simulink model "DIPC"  (R2015a)
settings: Solver=ode1  StartTime=0.0  StopTime=3.0  FixedStep=1e-3  RelTol=1e-3
values from neighbouring files (symbols this model uses):
  deltas = 300    [DIPCinit.m]
  deltav = 2000    [DIPCinit.m]
  ds = 300    [DIPCinit.m]
  dv = 5000    [DIPCinit.m]
  g = [0;0;0]    [DIPCinit.m]
  j0 = 1    [DIPCinit.m]
  j1 = 10    [DIPCinit.m]
  j2 = 10    [DIPCinit.m]
  j3 = 10    [DIPCinit.m]
  j4 = 10    [DIPCinit.m]
  jv = 1    [DIPCinit.m]
  kappas = 500    [DIPCinit.m]
  kappav = 2000    [DIPCinit.m]
  ks = 500    [DIPCinit.m]
  kv = 20000    [DIPCinit.m]
  m0 = 10    [DIPCinit.m]
  m1 = 10    [DIPCinit.m]
  m2 = 10    [DIPCinit.m]
  m3 = 10    [DIPCinit.m]
  m4 = 10    [DIPCinit.m]
  mv = 10    [DIPCinit.m]
libraries: aerolibutil x11, dspinverses x3, aerolibtransform2 x2, simulink x2
settings Model: CovSFcnEnable=off  Creator=Martin  LastModifiedBy=mangerer
settings OptimizationCC: BlockReduction=off  OptimizeBlockIOStorage=off  BufferReuse=off  GlobalBufferReuse=off  ExpressionFolding=off  LocalBlockOutputs=off
settings DebuggingCC: SolverPrmCheckMsg=warning

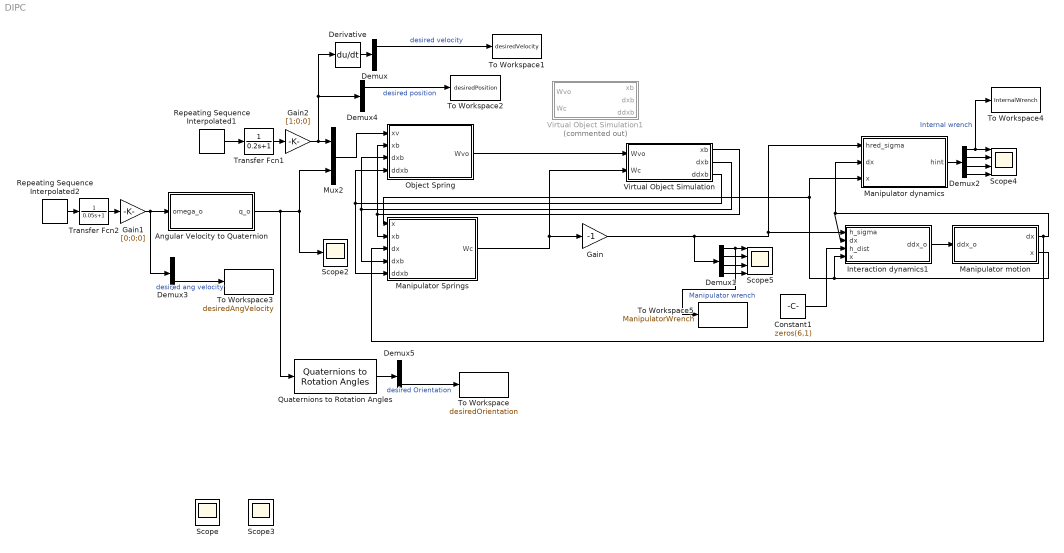
== system DIPC ==
  Angular Velocity to Quaternion : Subsystem
  Constant1 : Constant  Value=zeros(6,1)
  Demux{,3..5} (4 alike) : Demux  Outputs=3
  Demux1 : Demux
  Demux2 : Demux
  Derivative : Derivative
  Gain : Gain  Gain=-1
  Gain1 : Gain  Gain=[0;0;0]
  Gain2 : Gain  Gain=[1;0;0]
  Interaction dynamics1 : Subsystem
  Manipulator Springs : Subsystem
  Manipulator dynamics : Subsystem
  Manipulator motion : Subsystem
  Mux2 : Mux  Inputs=2
  Object Spring : Subsystem
  Quaternions to Rotation Angles : aerolibtransform2/Quaternions to Rotation Angles  rotationOrder=XYZ
  Repeating Sequence Interpolated1 : simulink/Sources/Repeating Sequence Interpolated  OutValues=[0 0 0.5 0.5 1 1 -0.5 -0.5 0 0].'  TimeValues=[0 0.1 0.14 0.9 0.96 1.8 1.95 2.4 2.6 3].'  LookUpMeth=Interpolation-Use End Values  tsamp=0.001  OutMin=[]  OutMax=[]  OutDataTypeStr=double  OutputDataTypeScalingMode=double  OutDataType=fixdt(0,8)  OutScaling=2^-10
  Repeating Sequence Interpolated2 : simulink/Sources/Repeating Sequence Interpolated  OutValues=[0 0 1 1 0 0].'  TimeValues=[0 0.1 1.5 2 2.5 3].'  LookUpMeth=Interpolation-Use End Values  tsamp=0.001  OutMin=[]  OutMax=[]  OutDataTypeStr=double  OutputDataTypeScalingMode=double  OutDataType=fixdt(0,8)  OutScaling=2^-10
  Scope{,3..5} (4 alike) : Scope  NumInputPorts=4
      Scope settings: Floating=on  ShowLegends=on  YMin=-0~0~-30~-0.04  YMax=1.5~1.25~30~0.07  SaveName=ScopeData5
      Scope3 settings: Floating=on  ShowLegends=on  YMin=-0.5~-6~-500~-2e-09  YMax=1~3~700~2.5e-09  SaveName=ScopeData12
      Scope4 settings: ShowLegends=on  YMin=-0.025~-0.025~-0.05~-0.05  YMax=0.05~0.05~0.025~0.025  SaveName=ScopeData6
      Scope5 settings: ShowLegends=on  YMin=-40~-40~-50~-50  YMax=60~60~30~30  SaveName=ScopeData11
  Scope2 : Scope
  To Workspace : ToWorkspace  VariableName=desiredOrientation  SaveFormat=Timeseries  SampleTime=-1
  To Workspace1 : ToWorkspace  VariableName=desiredVelocity  SaveFormat=Timeseries  SampleTime=-1
  To Workspace2 : ToWorkspace  VariableName=desiredPosition  SaveFormat=Timeseries  SampleTime=-1
  To Workspace3 : ToWorkspace  VariableName=desiredAngVelocity  SaveFormat=Timeseries  SampleTime=-1
  To Workspace4 : ToWorkspace  VariableName=InternalWrench  SaveFormat=Timeseries  SampleTime=-1
  To Workspace5 : ToWorkspace  VariableName=ManipulatorWrench  SaveFormat=Timeseries  SampleTime=-1
  Transfer Fcn1 : TransferFcn  Denominator=[0.2 1]
  Transfer Fcn2 : TransferFcn  Denominator=[0.05 1]
  Virtual Object Simulation : Subsystem
  Virtual Object Simulation1 : Subsystem  Commented=on
  wires:
  Object Spring/1(Wvo) -> Virtual Object Simulation/1(Wvo)
  Virtual Object Simulation/1(xb) -> Object Spring/2(xb), Manipulator Springs/2(xb)
  Manipulator Springs/1(Wc) -> Virtual Object Simulation/2(Wc), Gain/1
  Interaction dynamics1/1(ddx_o) -> Manipulator motion/1(ddx_o)
  Constant1/1 -> Interaction dynamics1/3(h_dist)
  Manipulator motion/1(dx) -> Manipulator Springs/3(dx), Manipulator dynamics/2(dx), Interaction dynamics1/2(dx)
  Manipulator motion/2(x) -> Manipulator dynamics/3(x), Manipulator Springs/1(x), Interaction dynamics1/4(x)
  Virtual Object Simulation/2(dxb) -> Manipulator Springs/4(dxb), Object Spring/3(dxb)
  Manipulator dynamics/1(hint) -> Demux2/1
  Demux2/2 -> Scope4/2
  Demux2/4 -> Scope4/4
  Demux2/3 -> Scope4/3
  Demux2/1 -> To Workspace4/1, Scope4/1  "Internal wrench"
  Repeating Sequence Interpolated1/1 -> Transfer Fcn1/1
  Transfer Fcn1/1 -> Gain2/1
  Gain2/1 -> Demux4/1, Derivative/1, Mux2/1
  Mux2/1 -> Object Spring/1(xv)
  Angular Velocity to Quaternion/1(q_o) -> Quaternions to Rotation Angles/1, Mux2/2, Scope2/1
  Repeating Sequence Interpolated2/1 -> Transfer Fcn2/1
  Transfer Fcn2/1 -> Gain1/1
  Gain1/1 -> Demux3/1, Angular Velocity to Quaternion/1(omega_o)
  Gain/1 -> Demux1/1, Manipulator dynamics/1(hred_sigma), Interaction dynamics1/1(h_sigma)
  Demux1/2 -> Scope5/2
  Demux1/4 -> Scope5/4
  Demux1/3 -> Scope5/3
  Demux1/1 -> To Workspace5/1, Scope5/1  "Manipulator wrench"
  Quaternions to Rotation Angles/1 -> Demux5/1
  Demux5/3 -> To Workspace/1  "desired Orientation"
  Demux3/3 -> To Workspace3/1  "desired ang velocity"
  Demux4/1 -> To Workspace2/1  "desired position"
  Demux/1 -> To Workspace1/1  "desired velocity"
  Derivative/1 -> Demux/1
  Virtual Object Simulation/3(ddxb) -> Object Spring/4(ddxb), Manipulator Springs/5(ddxb)

== system DIPC/Angular Velocity to Quaternion ==
  omega_o : Inport
  Constant : Constant  Value=0
  Gain : Gain  Gain=0.5
  Integrator : Integrator  InitialCondition=[1; 0; 0; 0]
  Mux : Mux  Inputs=2
  Quaternion Multiplication : aerolibutil/Quaternion Multiplication
  Scope : Scope
      settings: ShowLegends=on  SaveName=ScopeData9
  q_o : Outport
  wires:
  omega_o/1 -> Gain/1
  Gain/1 -> Mux/2
  Constant/1 -> Mux/1
  Quaternion Multiplication/1 -> Integrator/1
  Integrator/1 -> Quaternion Multiplication/2, q_o/1, Scope/1
  Mux/1 -> Quaternion Multiplication/1

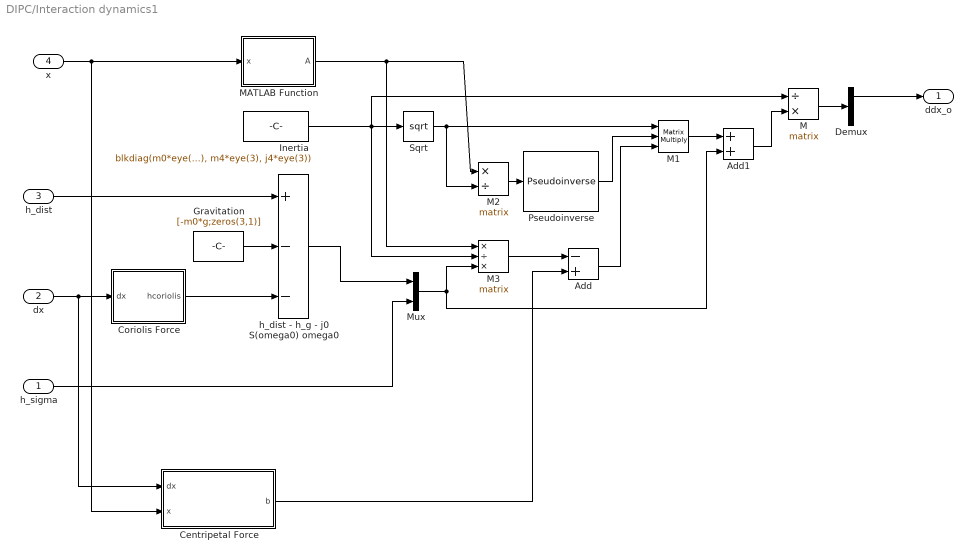
== system DIPC/Interaction dynamics1 ==
  h_sigma : Inport
  dx : Inport  Port=2
  h_dist : Inport  Port=3
  x : Inport  Port=4
  Add : Sum  Inputs=-+
  Add1 : Sum
  Centripetal Force : MATLAB Function  TreatAsAtomicUnit=on
  Coriolis Force : MATLAB Function  TreatAsAtomicUnit=on
  Demux : Demux  Outputs=5
  Gravitation : Constant  Value=[-m0*g;zeros(3,1)]
  Inertia : Constant  Value=blkdiag(m0*eye(3),j0*eye(3),m1*eye(3), j1*eye(3), m2*eye(3), j2*eye(3),m3*eye(3), j3*eye(3), m4*eye(3), j4*eye(3))
  M : Product  Inputs=/*  Multiplication=Matrix(*)
  M1 : Product  Inputs=***  Multiplication=Matrix(*)
  M2 : Product  Inputs=*/  Multiplication=Matrix(*)
  M3 : Product  Inputs=*/*  Multiplication=Matrix(*)
  MATLAB Function : MATLAB Function  TreatAsAtomicUnit=on
  Mux : Mux  Inputs=2
  Pseudoinverse : dspinverses/Pseudoinverse  wanterr=off
  Sqrt : Sqrt  SaturateOnIntegerOverflow=on
  "h_dist - h_g - j0 S(omega0) omega0 " : Sum  Inputs=+--
  ddx_o : Outport
  wires:
  h_dist/1 -> "h_dist - h_g - j0 S(omega0) omega0 "/1
  Gravitation/1 -> "h_dist - h_g - j0 S(omega0) omega0 "/2
  dx/1 -> Centripetal Force/1(dx), Coriolis Force/1(dx)
  Coriolis Force/1(hcoriolis) -> "h_dist - h_g - j0 S(omega0) omega0 "/3
  x/1 -> MATLAB Function/1(x), Centripetal Force/2(x)
  Inertia/1 -> M/1, M3/2, Sqrt/1
  Sqrt/1 -> M2/2, M1/1
  MATLAB Function/1(A) -> M3/1, M2/1
  M2/1 -> Pseudoinverse/1
  Pseudoinverse/1 -> M1/2
  Add/1 -> M1/3
  Centripetal Force/1(b) -> Add/2
  M3/1 -> Add/1
  Mux/1 -> Add1/2, M3/3
  "h_dist - h_g - j0 S(omega0) omega0 "/1 -> Mux/1
  h_sigma/1 -> Mux/2
  M/1 -> Demux/1
  Demux/1 -> ddx_o/1
  M1/1 -> Add1/1
  Add1/1 -> M/2

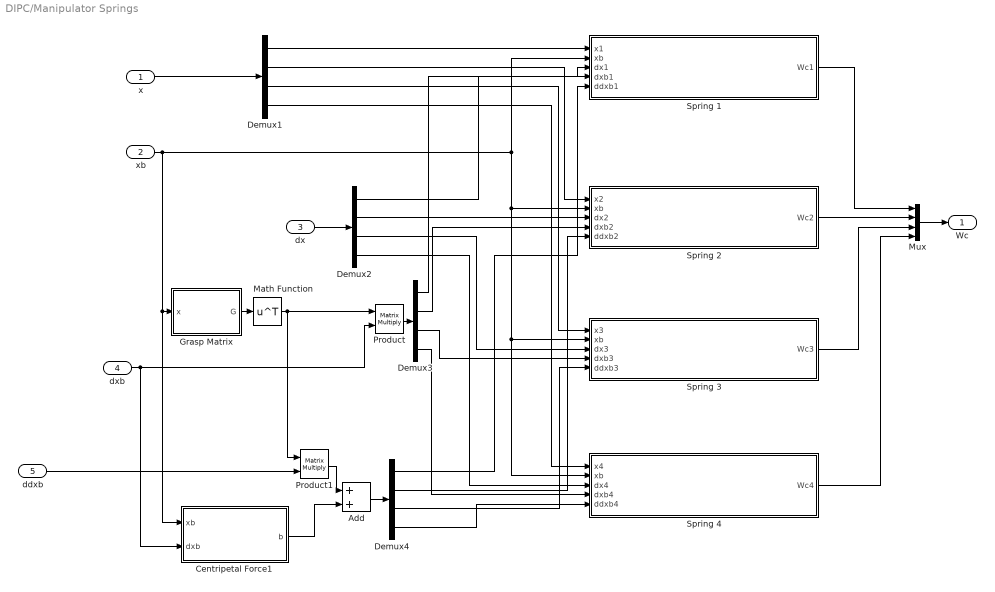
== system DIPC/Manipulator Springs ==
  x : Inport
  xb : Inport  Port=2
  dx : Inport  Port=3
  dxb : Inport  Port=4
  ddxb : Inport  Port=5
  Add : Sum
  Centripetal Force1 : MATLAB Function  TreatAsAtomicUnit=on
  Demux{1..4} (4 alike) : Demux
  Grasp Matrix : MATLAB Function  TreatAsAtomicUnit=on
  Math Function : Math  Operator=transpose  SaturateOnIntegerOverflow=on
  Mux : Mux
  Product : Product  Multiplication=Matrix(*)
  Product1 : Product  Multiplication=Matrix(*)
  Spring 1 : Subsystem
  Spring 2 : Subsystem
  Spring 3 : Subsystem
  Spring 4 : Subsystem
  Wc : Outport
  wires:
  Spring 1/1(Wc1) -> Mux/1
  Spring 2/1(Wc2) -> Mux/2
  Mux/1 -> Wc/1
  x/1 -> Demux1/1
  Spring 3/1(Wc3) -> Mux/3
  Spring 4/1(Wc4) -> Mux/4
  dx/1 -> Demux2/1
  Grasp Matrix/1(G) -> Math Function/1
  Math Function/1 -> Product/1, Product1/1
  dxb/1 -> Product/2, Centripetal Force1/2(dxb)
  Product/1 -> Demux3/1
  Demux1/1 -> Spring 1/1(x1)
  Demux1/2 -> Spring 2/1(x2)
  Demux1/3 -> Spring 3/1(x3)
  Demux1/4 -> Spring 4/1(x4)
  xb/1 -> Spring 1/2(xb), Spring 4/2(xb), Spring 3/2(xb), Spring 2/2(xb), Grasp Matrix/1(x), Centripetal Force1/1(xb)
  Demux2/1 -> Spring 1/3(dx1)
  Demux2/2 -> Spring 2/3(dx2)
  Demux2/3 -> Spring 3/3(dx3)
  Demux2/4 -> Spring 4/3(dx4)
  Demux3/1 -> Spring 1/4(dxb1)
  Demux3/2 -> Spring 2/4(dxb2)
  Demux3/3 -> Spring 3/4(dxb3)
  Demux3/4 -> Spring 4/4(dxb4)
  ddxb/1 -> Product1/2
  Centripetal Force1/1(b) -> Add/2
  Product1/1 -> Add/1
  Demux4/1 -> Spring 1/5(ddxb1)
  Demux4/2 -> Spring 2/5(ddxb2)
  Demux4/3 -> Spring 3/5(ddxb3)
  Demux4/4 -> Spring 4/5(ddxb4)
  Add/1 -> Demux4/1

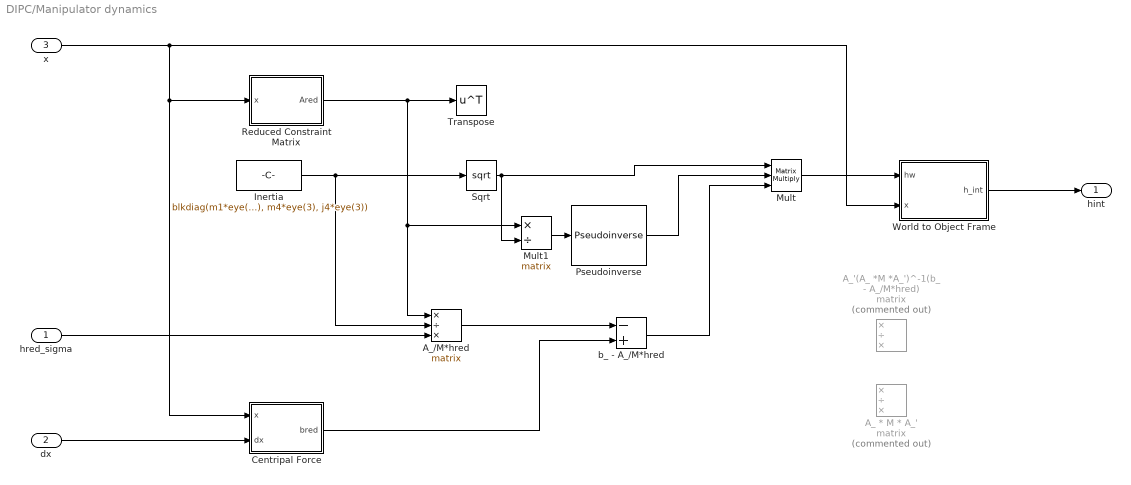
== system DIPC/Manipulator dynamics ==
  hred_sigma : Inport
  dx : Inport  Port=2
  x : Inport  Port=3
  A_ * M * A_' : Product  Commented=on  Inputs=*/*  Multiplication=Matrix(*)
  A_'(A_ *M *A_')^-1(b_ - A_/M*hred) : Product  Commented=on  Inputs=*/*  Multiplication=Matrix(*)
  A_/M*hred : Product  Inputs=*/*  Multiplication=Matrix(*)
  Centripal Force : MATLAB Function  TreatAsAtomicUnit=on
  Inertia : Constant  Value=blkdiag(m1*eye(3), j1*eye(3), m2*eye(3), j2*eye(3), m3*eye(3), j3*eye(3), m4*eye(3), j4*eye(3))
  Mult : Product  Inputs=***  Multiplication=Matrix(*)
  Mult1 : Product  Inputs=*/  Multiplication=Matrix(*)
  Pseudoinverse : dspinverses/Pseudoinverse  wanterr=off
  Reduced Constraint Matrix : MATLAB Function  TreatAsAtomicUnit=on
  Sqrt : Sqrt  SaturateOnIntegerOverflow=on
  Transpose : Math  Operator=transpose  SaturateOnIntegerOverflow=on
  World to Object Frame : MATLAB Function  TreatAsAtomicUnit=on
  b_ - A_/M*hred : Sum  Inputs=-+
  hint : Outport
  wires:
  Reduced Constraint Matrix/1(Ared) -> Transpose/1, A_/M*hred/1, Mult1/1
  Inertia/1 -> Sqrt/1, A_/M*hred/2
  dx/1 -> Centripal Force/2(dx)
  A_/M*hred/1 -> b_ - A_/M*hred/1
  hred_sigma/1 -> A_/M*hred/3
  World to Object Frame/1(h_int) -> hint/1
  x/1 -> Centripal Force/1(x), Reduced Constraint Matrix/1(x), World to Object Frame/2(x)
  Centripal Force/1(bred) -> b_ - A_/M*hred/2
  Mult/1 -> World to Object Frame/1(hw)
  b_ - A_/M*hred/1 -> Mult/3
  Sqrt/1 -> Mult1/2, Mult/1
  Mult1/1 -> Pseudoinverse/1
  Pseudoinverse/1 -> Mult/2

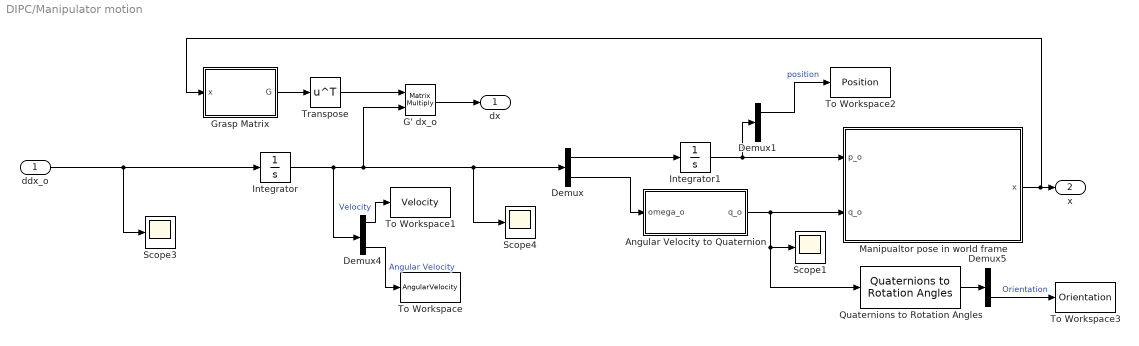
== system DIPC/Manipulator motion ==
  ddx_o : Inport
  Angular Velocity to Quaternion : Subsystem
  Demux : Demux  Outputs=2
  Demux1 : Demux  Outputs=3
  Demux4 : Demux  Outputs=6
  Demux5 : Demux  Outputs=3
  G' dx_o : Product  Multiplication=Matrix(*)
  Grasp Matrix : MATLAB Function  TreatAsAtomicUnit=on
  Integrator : Integrator  InitialCondition=zeros(6,1)
  Integrator1 : Integrator  InitialCondition=[0 0 0]'
  Manipualtor pose in world frame : MATLAB Function  TreatAsAtomicUnit=on
  Quaternions to Rotation Angles : aerolibtransform2/Quaternions to Rotation Angles  rotationOrder=XYZ
  Scope1 : Scope
      settings: SaveName=ScopeData13
  Scope3 : Scope
      settings: SaveName=ScopeData7
  Scope4 : Scope
      settings: SaveName=ScopeData16
  To Workspace : ToWorkspace  VariableName=AngularVelocity  SaveFormat=Timeseries  SampleTime=-1
  To Workspace1 : ToWorkspace  VariableName=Velocity  SaveFormat=Timeseries  SampleTime=-1
  To Workspace2 : ToWorkspace  VariableName=Position  SaveFormat=Timeseries  SampleTime=-1
  To Workspace3 : ToWorkspace  VariableName=Orientation  SaveFormat=Timeseries  SampleTime=-1
  Transpose : Math  Operator=transpose  SaturateOnIntegerOverflow=on
  dx : Outport
  x : Outport  Port=2
  wires:
  ddx_o/1 -> Scope3/1, Integrator/1
  Integrator/1 -> Demux4/1, G' dx_o/2, Scope4/1, Demux/1
  Grasp Matrix/1(G) -> Transpose/1
  Transpose/1 -> G' dx_o/1
  G' dx_o/1 -> dx/1
  Demux/2 -> Angular Velocity to Quaternion/1(omega_o)
  Demux/1 -> Integrator1/1
  Integrator1/1 -> Demux1/1, Manipualtor pose in world frame/1(p_o)
  Manipualtor pose in world frame/1(x) -> Grasp Matrix/1(x), x/1
  Angular Velocity to Quaternion/1(q_o) -> Scope1/1, Quaternions to Rotation Angles/1, Manipualtor pose in world frame/2(q_o)
  Demux4/1 -> To Workspace1/1  "Velocity"
  Demux4/6 -> To Workspace/1  "Angular Velocity"
  Quaternions to Rotation Angles/1 -> Demux5/1
  Demux5/3 -> To Workspace3/1  "Orientation"
  Demux1/1 -> To Workspace2/1  "position"

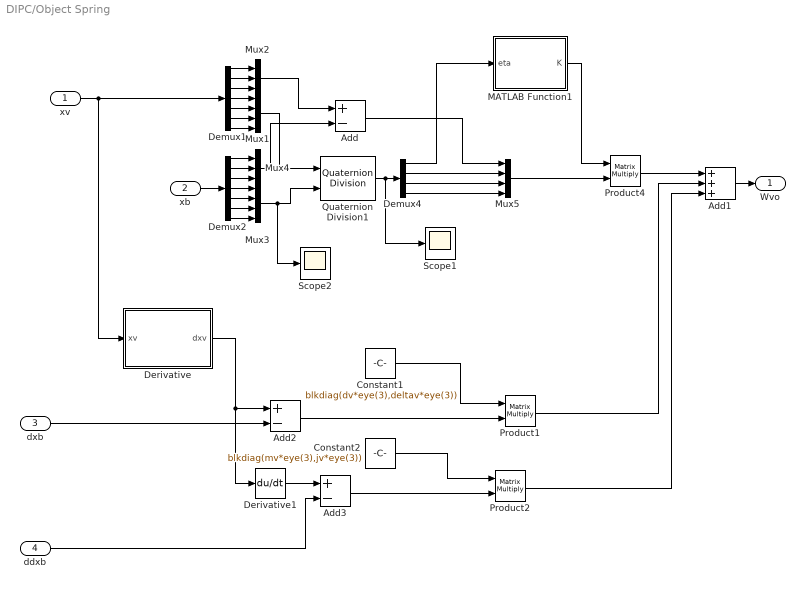
== system DIPC/Object Spring ==
  xv : Inport
  xb : Inport  Port=2
  dxb : Inport  Port=3
  ddxb : Inport  Port=4
  Add : Sum  Inputs=+-
  Add1 : Sum  Inputs=+++
  Add2 : Sum  Inputs=+-
  Add3 : Sum  Inputs=+-
  Constant1 : Constant  Value=blkdiag(dv*eye(3),deltav*eye(3))
  Constant2 : Constant  Value=blkdiag(mv*eye(3),jv*eye(3))
  Demux1 : Demux  Outputs=7
  Demux2 : Demux  Outputs=7
  Demux4 : Demux
  Derivative : Subsystem
  Derivative1 : Derivative
  MATLAB Function1 : MATLAB Function  TreatAsAtomicUnit=on
  Mux1 : Mux
  Mux2 : Mux  Inputs=3
  Mux3 : Mux
  Mux4 : Mux  Inputs=3
  Mux5 : Mux
  Product1 : Product  Multiplication=Matrix(*)
  Product2 : Product  Multiplication=Matrix(*)
  Product4 : Product  Multiplication=Matrix(*)
  Quaternion Division1 : aerolibutil/Quaternion Division
  Scope1 : Scope
      settings: SaveName=ScopeData3
  Scope2 : Scope
      settings: SaveName=ScopeData4
  Wvo : Outport
  wires:
  Add1/1 -> Wvo/1
  Product4/1 -> Add1/1
  Product1/1 -> Add1/2
  Constant1/1 -> Product1/1
  MATLAB Function1/1(K) -> Product4/1
  Demux4/1 -> MATLAB Function1/1(eta)
  Add/1 -> Mux5/1
  Demux4/2 -> Mux5/2
  Demux4/3 -> Mux5/3
  Demux4/4 -> Mux5/4
  Quaternion Division1/1 -> Scope1/1, Demux4/1
  Mux5/1 -> Product4/2
  xv/1 -> Derivative/1(xv), Demux1/1
  xb/1 -> Demux2/1
  Demux1/4 -> Mux1/1
  Demux1/5 -> Mux1/2
  Demux1/6 -> Mux1/3
  Demux1/7 -> Mux1/4
  Demux1/1 -> Mux2/1
  Demux1/2 -> Mux2/2
  Demux1/3 -> Mux2/3
  Mux1/1 -> Quaternion Division1/1
  Demux2/4 -> Mux3/1
  Demux2/5 -> Mux3/2
  Demux2/6 -> Mux3/3
  Demux2/7 -> Mux3/4
  Demux2/1 -> Mux4/1
  Demux2/2 -> Mux4/2
  Demux2/3 -> Mux4/3
  Mux4/1 -> Add/2
  Mux3/1 -> Scope2/1, Quaternion Division1/2
  Mux2/1 -> Add/1
  Add2/1 -> Product1/2
  Derivative/1(dxv) -> Derivative1/1, Add2/1
  dxb/1 -> Add2/2
  Derivative1/1 -> Add3/1
  Add3/1 -> Product2/2
  Constant2/1 -> Product2/1
  Product2/1 -> Add1/3
  ddxb/1 -> Add3/2

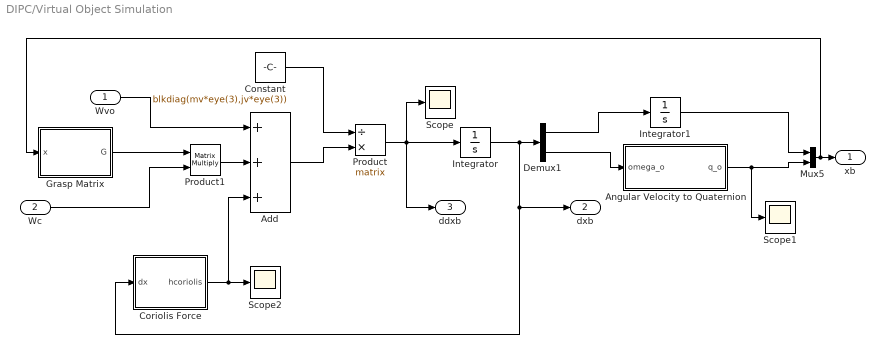
== system DIPC/Virtual Object Simulation ==
  Wvo : Inport
  Wc : Inport  Port=2
  Add : Sum  Inputs=+++
  Angular Velocity to Quaternion : Subsystem
  Constant : Constant  Value=blkdiag(mv*eye(3),jv*eye(3))
  Coriolis Force : MATLAB Function  TreatAsAtomicUnit=on
  Demux1 : Demux  Outputs=2
  Grasp Matrix : MATLAB Function  TreatAsAtomicUnit=on
  Integrator : Integrator  InitialCondition=zeros(6,1)
  Integrator1 : Integrator  InitialCondition=[0 0 0]'
  Mux5 : Mux  Inputs=2
  Product : Product  Inputs=/*  Multiplication=Matrix(*)
  Product1 : Product  Inputs=**  Multiplication=Matrix(*)
  Scope : Scope
  Scope1 : Scope
      settings: SaveName=ScopeData8
  Scope2 : Scope
      settings: YMin=-0.008  YMax=0.008  SaveName=ScopeData10
  xb : Outport
  dxb : Outport  Port=2
  ddxb : Outport  Port=3
  wires:
  Add/1 -> Product/2
  Constant/1 -> Product/1
  Product/1 -> ddxb/1, Scope/1, Integrator/1
  Integrator/1 -> Demux1/1, Coriolis Force/1(dx), dxb/1
  Demux1/2 -> Angular Velocity to Quaternion/1(omega_o)
  Demux1/1 -> Integrator1/1
  Integrator1/1 -> Mux5/1
  Angular Velocity to Quaternion/1(q_o) -> Scope1/1, Mux5/2
  Mux5/1 -> Grasp Matrix/1(x), xb/1
  Wvo/1 -> Add/1
  Product1/1 -> Add/2
  Grasp Matrix/1(G) -> Product1/1
  Wc/1 -> Product1/2
  Coriolis Force/1(hcoriolis) -> Scope2/1, Add/3

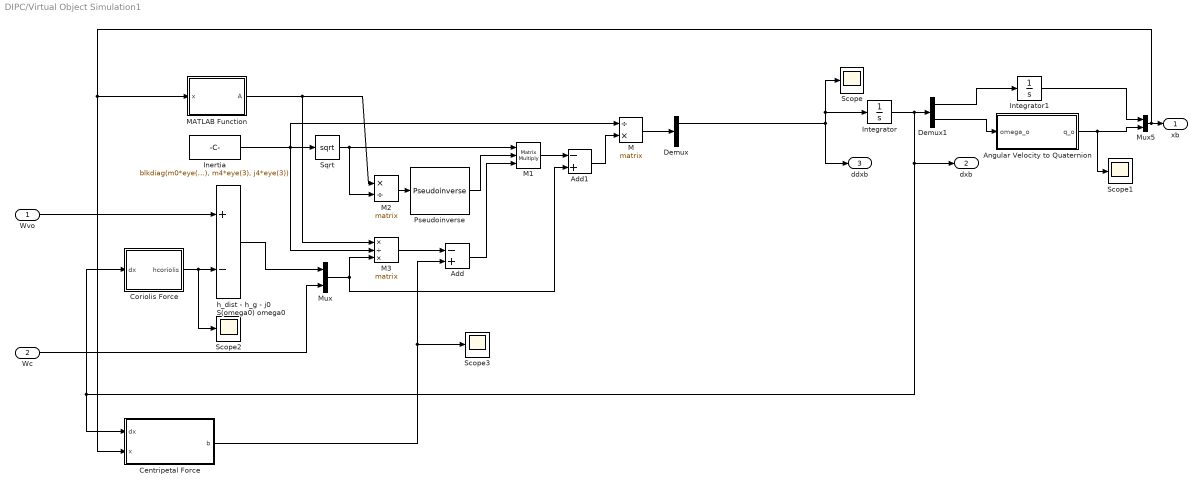
== system DIPC/Virtual Object Simulation1 ==
  Wvo : Inport
  Wc : Inport  Port=2
  Add : Sum  Inputs=-+
  Add1 : Sum  Inputs=-+
  Angular Velocity to Quaternion : Subsystem
  Centripetal Force : MATLAB Function  TreatAsAtomicUnit=on
  Coriolis Force : MATLAB Function  TreatAsAtomicUnit=on
  Demux : Demux  Outputs=5
  Demux1 : Demux  Outputs=2
  Inertia : Constant  Value=blkdiag(m0*eye(3),j0*eye(3),m1*eye(3), j1*eye(3), m2*eye(3), j2*eye(3),m3*eye(3), j3*eye(3), m4*eye(3), j4*eye(3))
  Integrator : Integrator  InitialCondition=zeros(6,1)
  Integrator1 : Integrator  InitialCondition=[0 0 0]'
  M : Product  Inputs=/*  Multiplication=Matrix(*)
  M1 : Product  Inputs=***  Multiplication=Matrix(*)
  M2 : Product  Inputs=*/  Multiplication=Matrix(*)
  M3 : Product  Inputs=*/*  Multiplication=Matrix(*)
  MATLAB Function : MATLAB Function  TreatAsAtomicUnit=on
  Mux : Mux  Inputs=2
  Mux5 : Mux  Inputs=2
  Pseudoinverse : dspinverses/Pseudoinverse  wanterr=off
  Scope{,1..3} (4 alike) : Scope
      Scope1 settings: SaveName=ScopeData8
      Scope2 settings: SaveName=ScopeData15
      Scope3 settings: YMin=-1  YMax=1  SaveName=ScopeData17
  Sqrt : Sqrt  SaturateOnIntegerOverflow=on
  "h_dist - h_g - j0 S(omega0) omega0 " : Sum  Inputs=+-
  xb : Outport
  dxb : Outport  Port=2
  ddxb : Outport  Port=3
  wires:
  Demux/1 -> Scope/1, Integrator/1, ddxb/1
  Integrator/1 -> Demux1/1, Coriolis Force/1(dx), Centripetal Force/1(dx), dxb/1
  Demux1/2 -> Angular Velocity to Quaternion/1(omega_o)
  Demux1/1 -> Integrator1/1
  Integrator1/1 -> Mux5/1
  Angular Velocity to Quaternion/1(q_o) -> Scope1/1, Mux5/2
  Wvo/1 -> "h_dist - h_g - j0 S(omega0) omega0 "/1
  Coriolis Force/1(hcoriolis) -> Scope2/1, "h_dist - h_g - j0 S(omega0) omega0 "/2
  Mux5/1 -> MATLAB Function/1(x), Centripetal Force/2(x), xb/1
  Inertia/1 -> M/1, M3/2, Sqrt/1
  Sqrt/1 -> M2/2, M1/1
  MATLAB Function/1(A) -> M3/1, M2/1
  M2/1 -> Pseudoinverse/1
  Pseudoinverse/1 -> M1/2
  Add/1 -> M1/3
  Centripetal Force/1(b) -> Scope3/1, Add/2
  M3/1 -> Add/1
  Mux/1 -> Add1/2, M3/3
  "h_dist - h_g - j0 S(omega0) omega0 "/1 -> Mux/1
  Wc/1 -> Mux/2
  M1/1 -> Add1/1
  Add1/1 -> M/2
  M/1 -> Demux/1

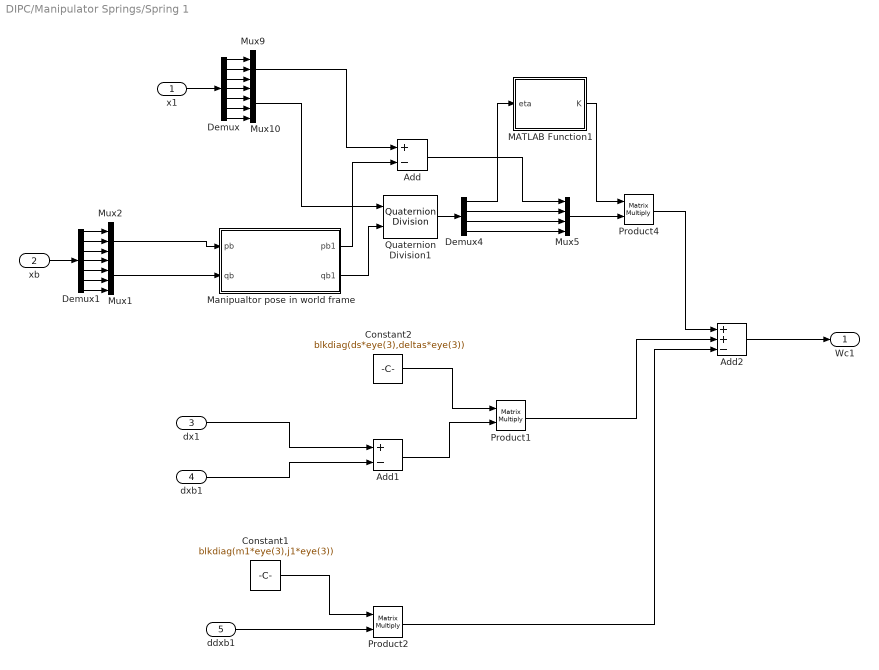
== system DIPC/Manipulator Springs/Spring 1 ==
  x1 : Inport
  xb : Inport  Port=2
  dx1 : Inport  Port=3
  dxb1 : Inport  Port=4
  ddxb1 : Inport  Port=5
  Add : Sum  Inputs=+-
  Add1 : Sum  Inputs=+-
  Add2 : Sum  Inputs=++-
  Constant1 : Constant  Value=blkdiag(m1*eye(3),j1*eye(3))
  Constant2 : Constant  Value=blkdiag(ds*eye(3),deltas*eye(3))
  Demux : Demux  Outputs=7
  Demux1 : Demux  Outputs=7
  Demux4 : Demux
  MATLAB Function1 : MATLAB Function  TreatAsAtomicUnit=on
  Manipualtor pose in world frame : MATLAB Function  TreatAsAtomicUnit=on
  Mux1 : Mux
  Mux10 : Mux
  Mux2 : Mux  Inputs=3
  Mux5 : Mux
  Mux9 : Mux  Inputs=3
  Product1 : Product  Multiplication=Matrix(*)
  Product2 : Product  Multiplication=Matrix(*)
  Product4 : Product  Multiplication=Matrix(*)
  Quaternion Division1 : aerolibutil/Quaternion Division
  Wc1 : Outport
  wires:
  Constant2/1 -> Product1/1
  Add2/1 -> Wc1/1
  x1/1 -> Demux/1
  Demux/1 -> Mux9/1
  Demux/2 -> Mux9/2
  Demux/3 -> Mux9/3
  Demux/4 -> Mux10/1
  Demux/5 -> Mux10/2
  Demux/6 -> Mux10/3
  Demux/7 -> Mux10/4
  MATLAB Function1/1(K) -> Product4/1
  Demux4/1 -> MATLAB Function1/1(eta)
  Add/1 -> Mux5/1
  Demux4/2 -> Mux5/2
  Demux4/3 -> Mux5/3
  Demux4/4 -> Mux5/4
  Quaternion Division1/1 -> Demux4/1
  Mux5/1 -> Product4/2
  Mux9/1 -> Add/1
  Manipualtor pose in world frame/1(pb1) -> Add/2
  Product4/1 -> Add2/1
  Mux10/1 -> Quaternion Division1/1
  Manipualtor pose in world frame/2(qb1) -> Quaternion Division1/2
  Product1/1 -> Add2/2
  dx1/1 -> Add1/1
  Add1/1 -> Product1/2
  dxb1/1 -> Add1/2
  Demux1/1 -> Mux2/1
  Demux1/2 -> Mux2/2
  Demux1/3 -> Mux2/3
  Demux1/4 -> Mux1/1
  Demux1/5 -> Mux1/2
  Demux1/6 -> Mux1/3
  Demux1/7 -> Mux1/4
  Mux2/1 -> Manipualtor pose in world frame/1(pb)
  Mux1/1 -> Manipualtor pose in world frame/2(qb)
  xb/1 -> Demux1/1
  Constant1/1 -> Product2/1
  ddxb1/1 -> Product2/2
  Product2/1 -> Add2/3

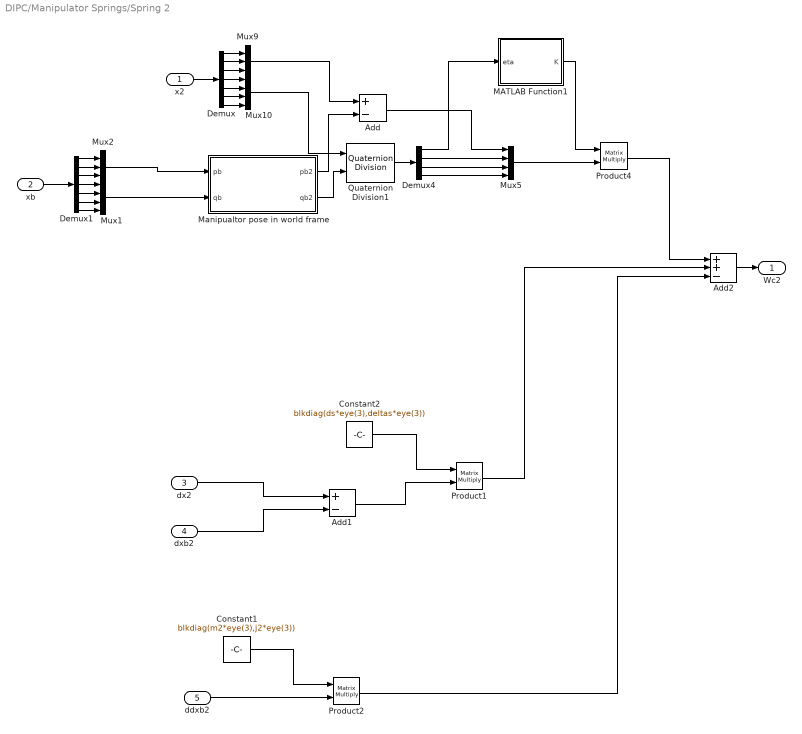
== system DIPC/Manipulator Springs/Spring 2 ==
  x2 : Inport
  xb : Inport  Port=2
  dx2 : Inport  Port=3
  dxb2 : Inport  Port=4
  ddxb2 : Inport  Port=5
  Add : Sum  Inputs=+-
  Add1 : Sum  Inputs=+-
  Add2 : Sum  Inputs=++-
  Constant1 : Constant  Value=blkdiag(m2*eye(3),j2*eye(3))
  Constant2 : Constant  Value=blkdiag(ds*eye(3),deltas*eye(3))
  Demux : Demux  Outputs=7
  Demux1 : Demux  Outputs=7
  Demux4 : Demux
  MATLAB Function1 : MATLAB Function  TreatAsAtomicUnit=on
  Manipualtor pose in world frame : MATLAB Function  TreatAsAtomicUnit=on
  Mux1 : Mux
  Mux10 : Mux
  Mux2 : Mux  Inputs=3
  Mux5 : Mux
  Mux9 : Mux  Inputs=3
  Product1 : Product  Multiplication=Matrix(*)
  Product2 : Product  Multiplication=Matrix(*)
  Product4 : Product  Multiplication=Matrix(*)
  Quaternion Division1 : aerolibutil/Quaternion Division
  Wc2 : Outport
  wires:
  Product1/1 -> Add2/2
  Constant2/1 -> Product1/1
  x2/1 -> Demux/1
  Demux/1 -> Mux9/1
  Demux/2 -> Mux9/2
  Demux/3 -> Mux9/3
  Demux/4 -> Mux10/1
  Demux/5 -> Mux10/2
  Demux/6 -> Mux10/3
  Demux/7 -> Mux10/4
  MATLAB Function1/1(K) -> Product4/1
  Demux4/1 -> MATLAB Function1/1(eta)
  Add/1 -> Mux5/1
  Demux4/2 -> Mux5/2
  Demux4/3 -> Mux5/3
  Demux4/4 -> Mux5/4
  Quaternion Division1/1 -> Demux4/1
  Mux5/1 -> Product4/2
  Mux9/1 -> Add/1
  Manipualtor pose in world frame/1(pb2) -> Add/2
  Manipualtor pose in world frame/2(qb2) -> Quaternion Division1/2
  Mux10/1 -> Quaternion Division1/1
  Add2/1 -> Wc2/1
  Product4/1 -> Add2/1
  Add1/1 -> Product1/2
  dx2/1 -> Add1/1
  dxb2/1 -> Add1/2
  xb/1 -> Demux1/1
  Demux1/1 -> Mux2/1
  Demux1/2 -> Mux2/2
  Demux1/3 -> Mux2/3
  Demux1/4 -> Mux1/1
  Demux1/5 -> Mux1/2
  Demux1/6 -> Mux1/3
  Demux1/7 -> Mux1/4
  Mux2/1 -> Manipualtor pose in world frame/1(pb)
  Mux1/1 -> Manipualtor pose in world frame/2(qb)
  Constant1/1 -> Product2/1
  ddxb2/1 -> Product2/2
  Product2/1 -> Add2/3

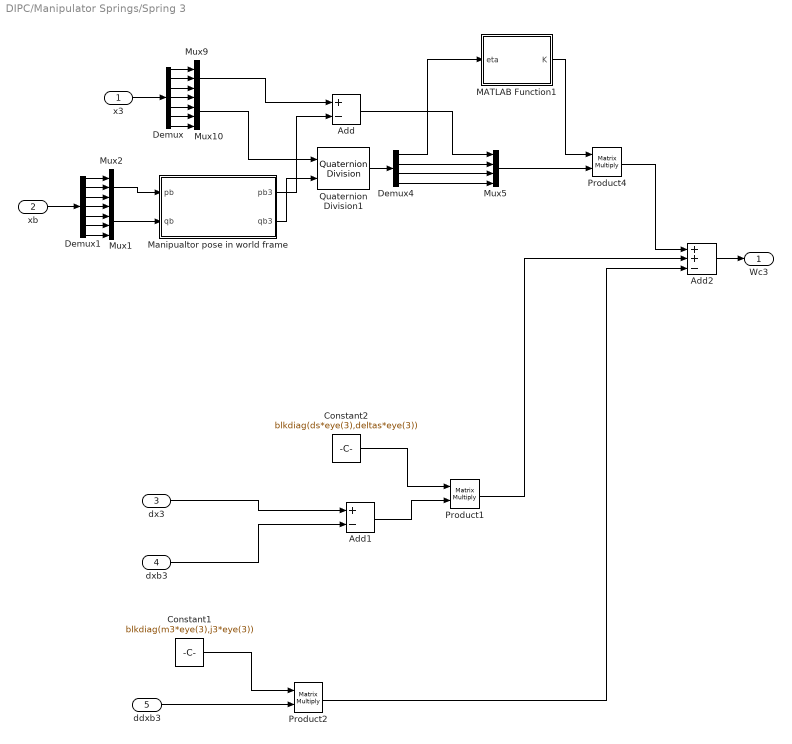
== system DIPC/Manipulator Springs/Spring 3 ==
  x3 : Inport
  xb : Inport  Port=2
  dx3 : Inport  Port=3
  dxb3 : Inport  Port=4
  ddxb3 : Inport  Port=5
  Add : Sum  Inputs=+-
  Add1 : Sum  Inputs=+-
  Add2 : Sum  Inputs=++-
  Constant1 : Constant  Value=blkdiag(m3*eye(3),j3*eye(3))
  Constant2 : Constant  Value=blkdiag(ds*eye(3),deltas*eye(3))
  Demux : Demux  Outputs=7
  Demux1 : Demux  Outputs=7
  Demux4 : Demux
  MATLAB Function1 : MATLAB Function  TreatAsAtomicUnit=on
  Manipualtor pose in world frame : MATLAB Function  TreatAsAtomicUnit=on
  Mux1 : Mux
  Mux10 : Mux
  Mux2 : Mux  Inputs=3
  Mux5 : Mux
  Mux9 : Mux  Inputs=3
  Product1 : Product  Multiplication=Matrix(*)
  Product2 : Product  Multiplication=Matrix(*)
  Product4 : Product  Multiplication=Matrix(*)
  Quaternion Division1 : aerolibutil/Quaternion Division
  Wc3 : Outport
  wires:
  Product1/1 -> Add2/2
  Constant2/1 -> Product1/1
  Add2/1 -> Wc3/1
  x3/1 -> Demux/1
  Demux/1 -> Mux9/1
  Demux/2 -> Mux9/2
  Demux/3 -> Mux9/3
  Demux/4 -> Mux10/1
  Demux/5 -> Mux10/2
  Demux/6 -> Mux10/3
  Demux/7 -> Mux10/4
  MATLAB Function1/1(K) -> Product4/1
  Demux4/1 -> MATLAB Function1/1(eta)
  Add/1 -> Mux5/1
  Demux4/2 -> Mux5/2
  Demux4/3 -> Mux5/3
  Demux4/4 -> Mux5/4
  Quaternion Division1/1 -> Demux4/1
  Mux5/1 -> Product4/2
  Product4/1 -> Add2/1
  Mux9/1 -> Add/1
  Manipualtor pose in world frame/1(pb3) -> Add/2
  Mux10/1 -> Quaternion Division1/1
  Manipualtor pose in world frame/2(qb3) -> Quaternion Division1/2
  Add1/1 -> Product1/2
  dx3/1 -> Add1/1
  dxb3/1 -> Add1/2
  xb/1 -> Demux1/1
  Demux1/1 -> Mux2/1
  Demux1/2 -> Mux2/2
  Demux1/3 -> Mux2/3
  Demux1/4 -> Mux1/1
  Demux1/5 -> Mux1/2
  Demux1/6 -> Mux1/3
  Demux1/7 -> Mux1/4
  Mux2/1 -> Manipualtor pose in world frame/1(pb)
  Mux1/1 -> Manipualtor pose in world frame/2(qb)
  Constant1/1 -> Product2/1
  ddxb3/1 -> Product2/2
  Product2/1 -> Add2/3

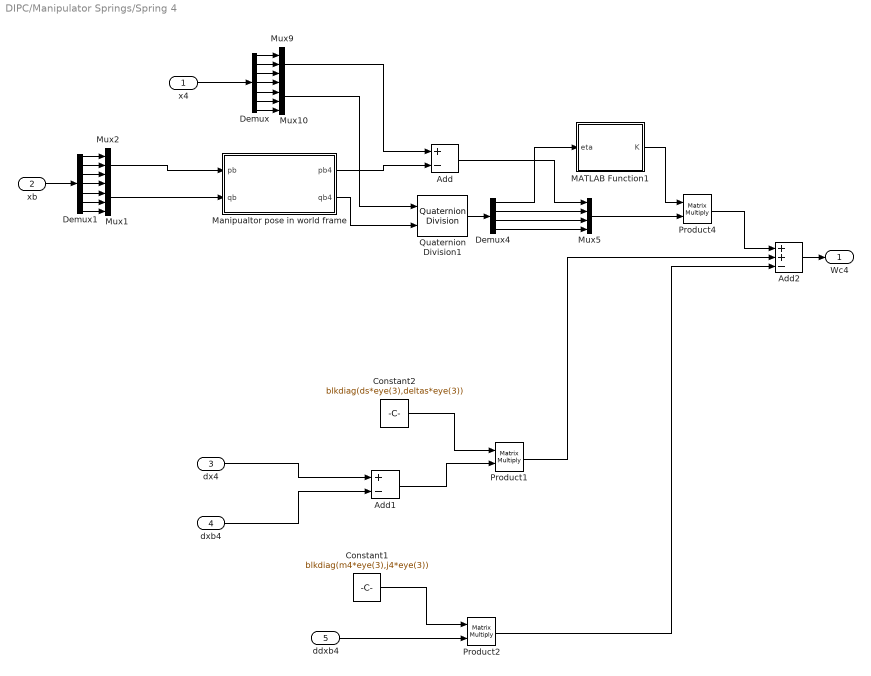
== system DIPC/Manipulator Springs/Spring 4 ==
  x4 : Inport
  xb : Inport  Port=2
  dx4 : Inport  Port=3
  dxb4 : Inport  Port=4
  ddxb4 : Inport  Port=5
  Add : Sum  Inputs=+-
  Add1 : Sum  Inputs=+-
  Add2 : Sum  Inputs=++-
  Constant1 : Constant  Value=blkdiag(m4*eye(3),j4*eye(3))
  Constant2 : Constant  Value=blkdiag(ds*eye(3),deltas*eye(3))
  Demux : Demux  Outputs=7
  Demux1 : Demux  Outputs=7
  Demux4 : Demux
  MATLAB Function1 : MATLAB Function  TreatAsAtomicUnit=on
  Manipualtor pose in world frame : MATLAB Function  TreatAsAtomicUnit=on
  Mux1 : Mux
  Mux10 : Mux
  Mux2 : Mux  Inputs=3
  Mux5 : Mux
  Mux9 : Mux  Inputs=3
  Product1 : Product  Multiplication=Matrix(*)
  Product2 : Product  Multiplication=Matrix(*)
  Product4 : Product  Multiplication=Matrix(*)
  Quaternion Division1 : aerolibutil/Quaternion Division
  Wc4 : Outport
  wires:
  Product1/1 -> Add2/2
  Constant2/1 -> Product1/1
  Add2/1 -> Wc4/1
  x4/1 -> Demux/1
  Demux/1 -> Mux9/1
  Demux/2 -> Mux9/2
  Demux/3 -> Mux9/3
  Demux/4 -> Mux10/1
  Demux/5 -> Mux10/2
  Demux/6 -> Mux10/3
  Demux/7 -> Mux10/4
  Demux4/2 -> Mux5/2
  Demux4/3 -> Mux5/3
  Demux4/4 -> Mux5/4
  Quaternion Division1/1 -> Demux4/1
  Mux5/1 -> Product4/2
  MATLAB Function1/1(K) -> Product4/1
  Demux4/1 -> MATLAB Function1/1(eta)
  Add/1 -> Mux5/1
  Mux9/1 -> Add/1
  Manipualtor pose in world frame/1(pb4) -> Add/2
  Mux10/1 -> Quaternion Division1/1
  Manipualtor pose in world frame/2(qb4) -> Quaternion Division1/2
  Product4/1 -> Add2/1
  Add1/1 -> Product1/2
  dx4/1 -> Add1/1
  dxb4/1 -> Add1/2
  xb/1 -> Demux1/1
  Demux1/1 -> Mux2/1
  Demux1/2 -> Mux2/2
  Demux1/3 -> Mux2/3
  Demux1/4 -> Mux1/1
  Demux1/5 -> Mux1/2
  Demux1/6 -> Mux1/3
  Demux1/7 -> Mux1/4
  Mux2/1 -> Manipualtor pose in world frame/1(pb)
  Mux1/1 -> Manipualtor pose in world frame/2(qb)
  Constant1/1 -> Product2/1
  ddxb4/1 -> Product2/2
  Product2/1 -> Add2/3

== system DIPC/Manipulator motion/Angular Velocity to Quaternion ==
  omega_o : Inport
  Constant : Constant  Value=0
  Gain : Gain  Gain=0.5
  Integrator : Integrator  InitialCondition=[1; 0; 0; 0]
  Mux : Mux  Inputs=2
  Quaternion Multiplication : aerolibutil/Quaternion Multiplication
  Scope : Scope
      settings: ShowLegends=on  SaveName=ScopeData9
  q_o : Outport
  wires:
  omega_o/1 -> Gain/1
  Gain/1 -> Mux/2
  Constant/1 -> Mux/1
  Quaternion Multiplication/1 -> Integrator/1
  Integrator/1 -> Quaternion Multiplication/2, q_o/1, Scope/1
  Mux/1 -> Quaternion Multiplication/1

== system DIPC/Object Spring/Derivative ==
  xv : Inport
  Demux3 : Demux  Outputs=7
  Demux5 : Demux
  Derivative : Derivative
  Derivative1 : Derivative
  Gain : Gain  Gain=2
  Mux : Mux  Inputs=3
  Mux6 : Mux
  Mux7 : Mux  Inputs=3
  Mux8 : Mux  Inputs=2
  Quaternion Conjugate : aerolibutil/Quaternion Conjugate
  Quaternion Multiplication : aerolibutil/Quaternion Multiplication
  Scope3 : Scope
      settings: ShowLegends=on  YMin=0  YMax=2  SaveName=ScopeData14
  T : Terminator
  dxv : Outport
  wires:
  Mux8/1 -> dxv/1
  xv/1 -> Demux3/1
  Demux5/1 -> T/1
  Demux3/1 -> Mux/1
  Demux3/2 -> Mux/2
  Demux3/3 -> Mux/3
  Demux3/4 -> Mux6/1
  Demux3/5 -> Mux6/2
  Demux3/6 -> Mux6/3
  Mux/1 -> Derivative/1
  Demux3/7 -> Mux6/4
  Gain/1 -> Scope3/1, Mux8/2
  Mux6/1 -> Quaternion Conjugate/1, Derivative1/1
  Derivative1/1 -> Quaternion Multiplication/1
  Quaternion Conjugate/1 -> Quaternion Multiplication/2
  Demux5/3 -> Mux7/2
  Quaternion Multiplication/1 -> Demux5/1
  Demux5/4 -> Mux7/3
  Mux7/1 -> Gain/1
  Demux5/2 -> Mux7/1
  Derivative/1 -> Mux8/1

== system DIPC/Virtual Object Simulation/Angular Velocity to Quaternion ==
  omega_o : Inport
  Constant : Constant  Value=0
  Gain : Gain  Gain=0.5
  Integrator : Integrator  InitialCondition=[1; 0; 0; 0]
  Mux : Mux  Inputs=2
  Quaternion Multiplication : aerolibutil/Quaternion Multiplication
  Scope : Scope
      settings: ShowLegends=on  SaveName=ScopeData9
  q_o : Outport
  wires:
  omega_o/1 -> Gain/1
  Gain/1 -> Mux/2
  Constant/1 -> Mux/1
  Quaternion Multiplication/1 -> Integrator/1
  Integrator/1 -> Quaternion Multiplication/2, q_o/1, Scope/1
  Mux/1 -> Quaternion Multiplication/1

== system DIPC/Virtual Object Simulation1/Angular Velocity to Quaternion ==
  omega_o : Inport
  Constant : Constant  Value=0
  Gain : Gain  Gain=0.5
  Integrator : Integrator  InitialCondition=[1; 0; 0; 0]
  Mux : Mux  Inputs=2
  Quaternion Multiplication : aerolibutil/Quaternion Multiplication
  Scope : Scope
      settings: ShowLegends=on  SaveName=ScopeData9
  q_o : Outport
  wires:
  omega_o/1 -> Gain/1
  Gain/1 -> Mux/2
  Constant/1 -> Mux/1
  Quaternion Multiplication/1 -> Integrator/1
  Integrator/1 -> Quaternion Multiplication/2, q_o/1, Scope/1
  Mux/1 -> Quaternion Multiplication/1

== matlab function DIPC/Manipulator Springs/Spring 1/Manipualtor pose in world frame ==
  data: pb input; qb input size=4; pb1 output; r parameter; qb1 output
function [pb1,qb1]= manipulatorpose(pb,qb,r)

pb1 = pb + quatrot(qb,r(1:3));
qb1 = qb;

== matlab function DIPC/Manipulator Springs/Spring 2/Manipualtor pose in world frame ==
  data: pb input; qb input size=4; pb2 output; r parameter; qb2 output
function [pb2,qb2]= manipulatorpose(pb,qb,r)

pb2 = pb + quatrot(qb,r(4:6));
qb2 = qb;

== matlab function DIPC/Manipulator Springs/Spring 3/Manipualtor pose in world frame ==
  data: pb input; qb input size=4; pb3 output; r parameter; qb3 output
function [pb3,qb3]= manipulatorpose(pb,qb,r)

pb3 = pb + quatrot(qb,r(7:9));
qb3 = qb;

== matlab function DIPC/Manipulator Springs/Spring 4/Manipualtor pose in world frame ==
  data: pb input; qb input size=4; pb4 output; r parameter; qb4 output
function [pb4,qb4]= manipulatorpose(pb,qb,r)

pb4 = pb + quatrot(qb,r(10:12));
qb4 = qb;

== matlab function DIPC/Interaction dynamics1/MATLAB Function ==
  data: r parameter; A output; x input
function A = ConstraintMatrix(r,x)
A = [-eye(3) skew_sm(quatrot(x(4:7),r(1:3))) eye(3) zeros(3,21);
        zeros(3) -eye(3) zeros(3) eye(3) zeros(3,18);
        -eye(3) skew_sm(quatrot(x(4:7),r(4:6))) zeros(3,6) eye(3) zeros(3,15);
        zeros(3) -eye(3) zeros(3,9) eye(3) zeros(3,12);
        -eye(3) skew_sm(quatrot(x(4:7),r(7:9))) zeros(3,12) eye(3) zeros(3,9);
        zeros(3) -eye(3) zeros(3,15) eye(3) zeros(3,6);
        -eye(3) skew_sm(quatrot(x(4:7),r(10:12))) zeros(3,18) eye(3) zeros(3);
        zeros(3) -eye(3) zeros(3,21) eye(3)];

== matlab function DIPC/Interaction dynamics1/Centripetal Force ==
  data: dx input; b output; r parameter; x input
function b = centripetalforce(dx,r,x)
b = [skew_sm(dx(4:6))*skew_sm(dx(4:6))*quatrot(x(4:7),r(1:3));
     zeros(3,1);
     skew_sm(dx(4:6))*skew_sm(dx(4:6))*quatrot(x(4:7),r(4:6));
     zeros(3,1);
     skew_sm(dx(4:6))*skew_sm(dx(4:6))*quatrot(x(4:7),r(7:9));
     zeros(3,1);
     skew_sm(dx(4:6))*skew_sm(dx(4:6))*quatrot(x(4:7),r(10:12));
     zeros(3,1)];

== matlab function DIPC/Interaction dynamics1/Coriolis Force ==
  data: dx input; hcoriolis output; j0 parameter; m0 parameter
function hcoriolis = CoriolisForce(dx,j0,m0)
hcoriolis = [m0*skew_sm(dx(4:6))*dx(1:3);
        j0*skew_sm(dx(4:6))*dx(4:6)];

== matlab function DIPC/Manipulator Springs/Spring 1/MATLAB Function1 ==
  data: eta input; K output; ks parameter; kappas parameter
function K = stiffness(eta,ks,kappas)
K = blkdiag(ks*eye(3),2*eta*kappas*eye(3));

== matlab function DIPC/Manipulator Springs/Spring 2/MATLAB Function1 ==
  data: eta input; K output; ks parameter; kappas parameter
function K = stiffness(eta,ks,kappas)
K = blkdiag(ks*eye(3),2*eta*kappas*eye(3));

== matlab function DIPC/Manipulator Springs/Spring 3/MATLAB Function1 ==
  data: eta input; K output; ks parameter; kappas parameter
function K = stiffness(eta,ks,kappas)
K = blkdiag(ks*eye(3),2*eta*kappas*eye(3));

== matlab function DIPC/Manipulator Springs/Spring 4/MATLAB Function1 ==
  data: eta input; K output; ks parameter; kappas parameter
function K = stiffness(eta,ks,kappas)
K = blkdiag(ks*eye(3),2*eta*kappas*eye(3));

== matlab function DIPC/Virtual Object Simulation/Grasp Matrix ==
  data: r parameter; G output; x input
function G = GraspMatrix(r,x)
G = [eye(3) zeros(3) eye(3) zeros(3) eye(3) zeros(3) eye(3) zeros(3);
    skew_sm(quatrot(x(4:7),r(1:3))) eye(3) skew_sm(quatrot(x(4:7),r(4:6))) eye(3) skew_sm(quatrot(x(4:7),r(7:9))) eye(3) skew_sm(quatrot(x(4:7),r(10:12))) eye(3)];

== matlab function DIPC/Virtual Object Simulation/Coriolis Force ==
  data: dx input; hcoriolis output; j0 parameter; m0 parameter
function hcoriolis = CoriolisForce(dx,j0,m0)
hcoriolis = [m0*skew_sm(dx(4:6))*dx(1:3);
        j0*skew_sm(dx(4:6))*dx(4:6)];

== matlab function DIPC/Virtual Object Simulation1/Centripetal Force ==
  data: dx input size=6; b output; r parameter; x input size=7
function b = centripetalforce(dx,r,x)
b = [skew_sm(dx(4:6))*skew_sm(dx(4:6))*quatrot(x(4:7),r(1:3));
     zeros(3,1);
     skew_sm(dx(4:6))*skew_sm(dx(4:6))*quatrot(x(4:7),r(4:6));
     zeros(3,1);
     skew_sm(dx(4:6))*skew_sm(dx(4:6))*quatrot(x(4:7),r(7:9));
     zeros(3,1);
     skew_sm(dx(4:6))*skew_sm(dx(4:6))*quatrot(x(4:7),r(10:12));
     zeros(3,1)];

== matlab function DIPC/Virtual Object Simulation1/Coriolis Force ==
  data: dx input; hcoriolis output; j0 parameter; m0 parameter
function hcoriolis = CoriolisForce(dx,j0,m0)
hcoriolis = [m0*skew_sm(dx(4:6))*dx(1:3);
        j0*skew_sm(dx(4:6))*dx(4:6)];

== matlab function DIPC/Virtual Object Simulation1/MATLAB Function ==
  data: r parameter; A output; x input
function A = ConstraintMatrix(r,x)
A = [-eye(3) skew_sm(quatrot(x(4:7),r(1:3))) eye(3) zeros(3,21);
        zeros(3) -eye(3) zeros(3) eye(3) zeros(3,18);
        -eye(3) skew_sm(quatrot(x(4:7),r(4:6))) zeros(3,6) eye(3) zeros(3,15);
        zeros(3) -eye(3) zeros(3,9) eye(3) zeros(3,12);
        -eye(3) skew_sm(quatrot(x(4:7),r(7:9))) zeros(3,12) eye(3) zeros(3,9);
        zeros(3) -eye(3) zeros(3,15) eye(3) zeros(3,6);
        -eye(3) skew_sm(quatrot(x(4:7),r(10:12))) zeros(3,18) eye(3) zeros(3);
        zeros(3) -eye(3) zeros(3,21) eye(3)];

== matlab function DIPC/Manipulator Springs/Grasp Matrix ==
  data: r parameter; G output; x input
function G = GraspMatrix(r,x)
G = [eye(3) zeros(3) eye(3) zeros(3) eye(3) zeros(3) eye(3) zeros(3);
    skew_sm(quatrot(x(4:7),r(1:3))) eye(3) skew_sm(quatrot(x(4:7),r(4:6))) eye(3) skew_sm(quatrot(x(4:7),r(7:9))) eye(3) skew_sm(quatrot(x(4:7),r(10:12))) eye(3)];

== matlab function DIPC/Manipulator Springs/Centripetal Force1 ==
  data: xb input; dxb input; b output; r parameter
function b = centripetalforce(xb,dxb,r)
b = [skew_sm(dxb(4:6))*skew_sm(dxb(4:6))*quatrot(xb(4:7),r(1:3));
     zeros(3,1);
     skew_sm(dxb(4:6))*skew_sm(dxb(4:6))*quatrot(xb(4:7),r(4:6));
     zeros(3,1);
     skew_sm(dxb(4:6))*skew_sm(dxb(4:6))*quatrot(xb(4:7),r(7:9));
     zeros(3,1);
     skew_sm(dxb(4:6))*skew_sm(dxb(4:6))*quatrot(xb(4:7),r(10:12));
     zeros(3,1)];

== matlab function DIPC/Object Spring/MATLAB Function1 ==
  data: eta input; K output; kv parameter; kappav parameter
function K = stiffness(eta,kv,kappav)
K = blkdiag(kv*eye(3),2*eta*kappav*eye(3));

== matlab function DIPC/Manipulator dynamics/Reduced Constraint Matrix ==
  data: r parameter; Ared output; x input
function Ared = ReducedConstraintMAtrix(r,x)
Ared = [-eye(3) skew_sm(quatrot(x(4:7),r(4:6)-r(1:3))) eye(3) zeros(3,15);
        zeros(3) -eye(3) zeros(3) eye(3) zeros(3,12);
        -eye(3) skew_sm(quatrot(x(4:7),r(7:9)-r(1:3))) zeros(3,6) eye(3) zeros(3,9);
        zeros(3) -eye(3) zeros(3,9) eye(3) zeros(3,6);
        -eye(3) skew_sm(quatrot(x(4:7),r(10:12)-r(1:3))) zeros(3,12) eye(3) zeros(3);
        zeros(3) -eye(3) zeros(3,15) eye(3)];

== matlab function DIPC/Manipulator dynamics/Centripal Force ==
  data: r parameter; x input; bred output; dx input
function bred = ReducedCentripetalvector(r,x,dx)
bred = [skew_sm(dx(4:6))*skew_sm(dx(4:6))*quatrot(x(4:7),(r(4:6)-r(1:3)));
        zeros(3,1);
        skew_sm(dx(4:6))*skew_sm(dx(4:6))*quatrot(x(4:7),(r(7:9)-r(1:3)));
        zeros(3,1);
        skew_sm(dx(4:6))*skew_sm(dx(4:6))*quatrot(x(4:7),(r(10:12)-r(1:3)));
        zeros(3,1)];

== matlab function DIPC/Manipulator motion/Grasp Matrix ==
  data: r parameter; G output; x input
function G = GraspMatrix(r,x)
G = [eye(3) zeros(3) eye(3) zeros(3) eye(3) zeros(3) eye(3) zeros(3);
    skew_sm(quatrot(x(4:7),r(1:3))) eye(3) skew_sm(quatrot(x(4:7),r(4:6))) eye(3) skew_sm(quatrot(x(4:7),r(7:9))) eye(3) skew_sm(quatrot(x(4:7),r(10:12))) eye(3)];

== matlab function DIPC/Manipulator motion/Manipualtor pose in world frame ==
  data: p_o input; q_o input size=4; x output; r parameter
function x = manipulatorpose(p_o,q_o,r)

x = [p_o + quatrot(q_o,r(1:3));
        q_o;
        p_o + quatrot(q_o,r(4:6));
        q_o;
        p_o + quatrot(q_o,r(7:9));
        q_o;
        p_o + quatrot(q_o,r(10:12));
        q_o ];

== matlab function DIPC/Manipulator dynamics/World to Object Frame ==
  data: hw input; x input; h_int output
function h_int = inertial2objectFrame(hw,x)

h_int = [quatrot(quatconj(x(4:7)')',hw(1:3));
         hw(4:6);%quatrot(quatconj(x(4:7)')',hw(4:6));
         quatrot(quatconj(x(4:7)')',hw(7:9));
         hw(10:12);%quatrot(quatconj(x(4:7)')',hw(10:12));
         quatrot(quatconj(x(4:7)')',hw(13:15));
         hw(16:18);%quatrot(quatconj(x(4:7)')',hw(16:18));
         quatrot(quatconj(x(4:7)')',hw(19:21));
         hw(22:24)];%quatrot(quatconj(x(4:7)')',hw(22:24));];
